simulink model "Task3"  (R2022a)
settings: Solver=FixedStepAuto  StartTime=0.0  StopTime=1.2  FixedStep=0.000001  RelTol=1e-3
values from neighbouring files (symbols this model uses):
  J_motor = 0.000610871894223    [var_10.mat]
  L_phase = 0.00332259990587    [var_10.mat]
  M_nom = 0.61236365542    [var_10.mat]
  psi = 0.0961787034043    [var_10.mat]
  R_phase = 0.753894801324    [var_10.mat]
  U_nom = 48    [var_10.mat]
undefined symbols (not defined in the file or in its folder): Kd_PID, Ki_PID, Kp_PID, T_delta
settings Model: Creator=Family  LastModifiedBy=Family

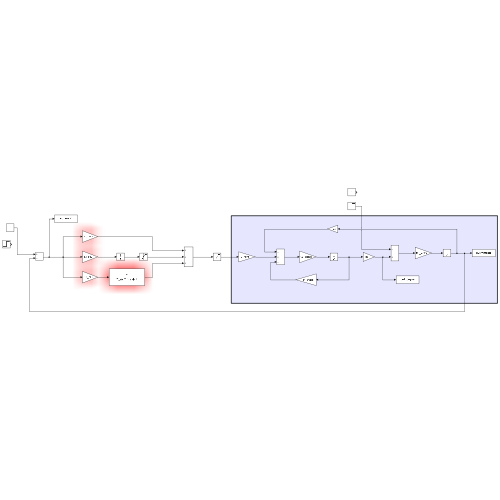
[thumbnail: Simulink's stored preview of the top-level diagram]
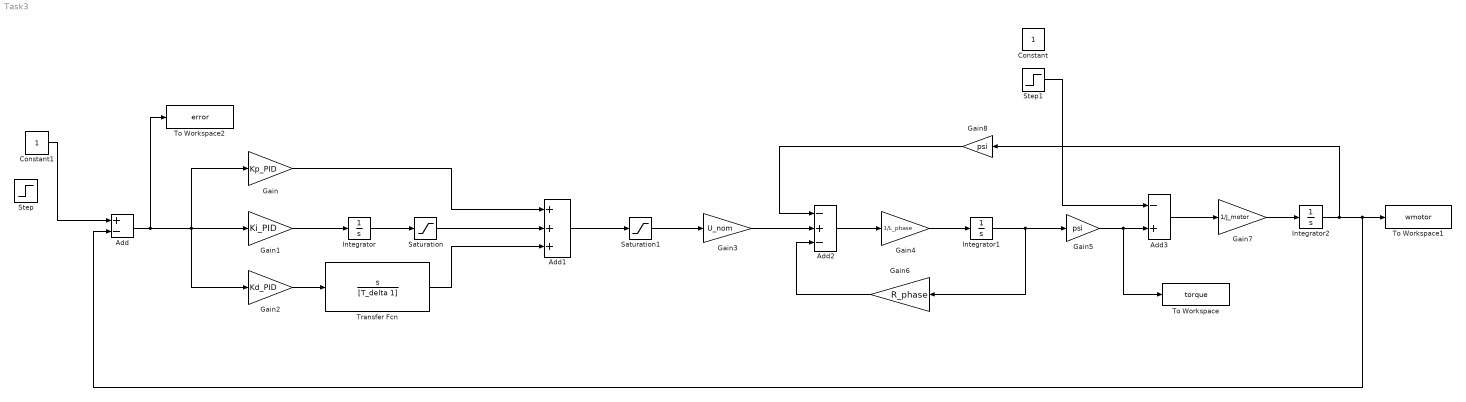
== system Task3 ==
  Add : Sum  Inputs=+-
  Add1 : Sum  Inputs=+++
  Add2 : Sum  Inputs=-+-
  Add3 : Sum  Inputs=-+
  Constant : Constant
  Constant1 : Constant
  Gain : Gain  Gain=Kp_PID
  Gain1 : Gain  Gain=Ki_PID
  Gain2 : Gain  Gain=Kd_PID
  Gain3 : Gain  Gain=U_nom
  Gain4 : Gain  Gain=1/L_phase
  Gain5 : Gain  Gain=psi
  Gain6 : Gain  Gain=R_phase
  Gain7 : Gain  Gain=1/J_motor
  Gain8 : Gain  Gain=psi
  Integrator : Integrator
  Integrator1 : Integrator
  Integrator2 : Integrator
  Saturation : Saturate  UpperLimit=1  LowerLimit=-1
  Saturation1 : Saturate  UpperLimit=1  LowerLimit=-1
  Step : Step  SampleTime=0.00001
  Step1 : Step  Before=0.5 * M_nom  After=M_nom  SampleTime=0
  To Workspace : ToWorkspace  VariableName=torque  SaveFormat=Timeseries  SampleTime=0.00001
  To Workspace1 : ToWorkspace  VariableName=wmotor  SaveFormat=Timeseries  SampleTime=0.00001
  To Workspace2 : ToWorkspace  VariableName=error  SaveFormat=Timeseries  SampleTime=0.00001
  Transfer Fcn : TransferFcn  Numerator=[1 0]  Denominator=[T_delta 1]
  wires:
  Gain/1 -> Add1/1
  Gain1/1 -> Integrator/1
  Gain2/1 -> Transfer Fcn/1
  Integrator/1 -> Saturation/1
  Saturation/1 -> Add1/2
  Add1/1 -> Saturation1/1
  Transfer Fcn/1 -> Add1/3
  Add/1 -> Gain/1, Gain2/1, Gain1/1, To Workspace2/1
  Add3/1 -> Gain7/1
  Integrator2/1 -> Add/2, To Workspace1/1, Gain8/1
  Gain7/1 -> Integrator2/1
  Step1/1 -> Add3/1
  Gain6/1 -> Add2/3
  Gain5/1 -> To Workspace/1, Add3/2
  Gain4/1 -> Integrator1/1
  Add2/1 -> Gain4/1
  Gain3/1 -> Add2/2
  Integrator1/1 -> Gain6/1, Gain5/1
  Gain8/1 -> Add2/1
  Saturation1/1 -> Gain3/1
  Constant1/1 -> Add/1
